simulink model "FPA_wired_subsystem_template"  (Simulink 7.5)
settings: Solver=ode45  StartTime=0.0  StopTime=10.0  RelTol=1e-3
undefined symbols (not defined in the file): slDataTypeAndScale, X0
settings Model: Creator=cliu  LastModifiedBy=cliu
settings DebuggingCC: StrictBusMsg=Warning

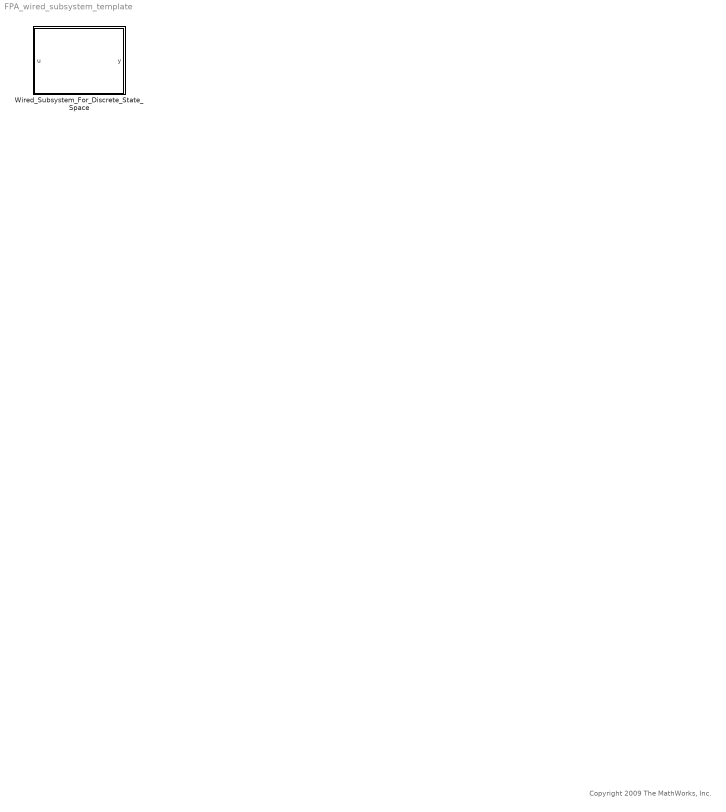
== system FPA_wired_subsystem_template ==
  note: Copyright 2009 The MathWorks, Inc.
  Wired_Subsystem_For_Discrete_State_Space : Subsystem

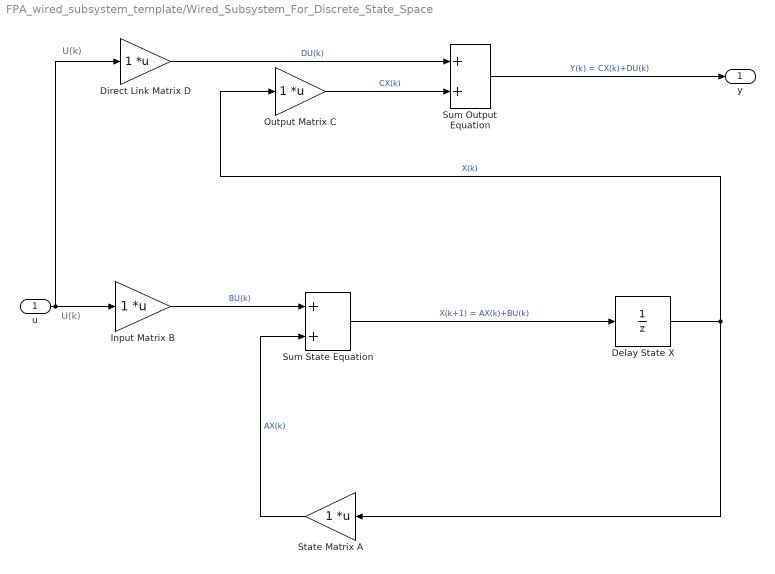
== system FPA_wired_subsystem_template/Wired_Subsystem_For_Discrete_State_Space ==
  note: U(k)
  note: U(k)
  u : Inport  OutDataType=fixdt(1, 16)  OutScaling=2^0
  Delay State X : UnitDelay  DisableCoverage=on  X0=X0  SampleTime=-1
      settings: AttributesFormatString=%<Description>
  Direct Link Matrix D : Gain  DisableCoverage=on  Multiplication=Matrix(K*u) (u vector)  ParameterDataType=sint(8)  ParameterScalingMode=Use specified scaling  ParameterScaling=1  OutDataType=sint(8)  OutScaling=1  OutDataTypeStr=Inherit: Inherit via back propagation
      settings: AttributesFormatString=%<Description>
  Input Matrix B : Gain  DisableCoverage=on  Multiplication=Matrix(K*u) (u vector)  ParameterDataType=sint(8)  ParameterScalingMode=Use specified scaling  ParameterScaling=1  OutDataType=sint(8)  OutScaling=1  OutDataTypeStr=Inherit: Inherit via back propagation
      settings: AttributesFormatString=%<Description>
  Output Matrix C : Gain  DisableCoverage=on  Multiplication=Matrix(K*u) (u vector)  ParameterDataType=sint(8)  ParameterScalingMode=Use specified scaling  ParameterScaling=1  OutDataType=sint(8)  OutScaling=1  OutDataTypeStr=Inherit: Inherit via back propagation
      settings: AttributesFormatString=%<Description>
  State Matrix A : Gain  DisableCoverage=on  Multiplication=Matrix(K*u) (u vector)  ParameterDataType=sint(8)  ParameterScalingMode=Use specified scaling  ParameterScaling=1  OutDataType=sint(8)  OutScaling=1  OutDataTypeStr=Inherit: Inherit via back propagation
      settings: AttributesFormatString=%<Description>
  Sum Output Equation : Sum  DisableCoverage=on  OutDataType=slDataTypeAndScale(('InternalDataType'),('OutputEqScaling'))
      settings: AttributesFormatString=%<Description>
  Sum State Equation : Sum  DisableCoverage=on  OutDataType=slDataTypeAndScale(('InternalDataType'),('StateEqScaling'))
      settings: AttributesFormatString=%<Description>
  y : Outport  OutDataType=fixdt(1, 16)  OutScaling=2^0  InitialOutput=0
  wires:
  State Matrix A/1 -> Sum State Equation/2  "AX(k)"
  u/1 -> Input Matrix B/1, Direct Link Matrix D/1
  Input Matrix B/1 -> Sum State Equation/1  "BU(k)"
  Sum State Equation/1 -> Delay State X/1  "X(k+1) = AX(k)+BU(k)"
  Delay State X/1 -> State Matrix A/1, Output Matrix C/1  "X(k)"
  Output Matrix C/1 -> Sum Output Equation/2  "CX(k)"
  Direct Link Matrix D/1 -> Sum Output Equation/1  "DU(k)"
  Sum Output Equation/1 -> y/1  "Y(k) = CX(k)+DU(k)"
